simulink model "Forward_and_inverse_Both"  (R2024b)
settings: Solver=VariableStepAuto  StartTime=0.0  StopTime=7  MaxStep=0.005  RelTol=1e-3
model workspace: external: MATLAB File D:\OneDrive - itc.edu.kh\V4_robot_arm\Import_arm6\Test_Assembly_DataFile.m (data not in the file)
values from neighbouring files (symbols this model uses):
  Reach_max = max(REACH_MAX)    [Workspace_sample.m]
  Reach_min = max(REACH_MIN)    [Workspace_sample.m]
undefined symbols (not defined in the file or in its folder): DiscIntNeverNeededParam, initialPose, maxAngularAcc, maxAngularVel, maxLinearAcc, maxLinearVel, poseTol, smiData, Ts, wps1, X, Y, Z
libraries: sm_lib x140, nesl_utility x52, stmnucleolib x12, simulink x4, vrlib x2, vexcommonlib x2, robotcorelib x2
(part 3 of 6)

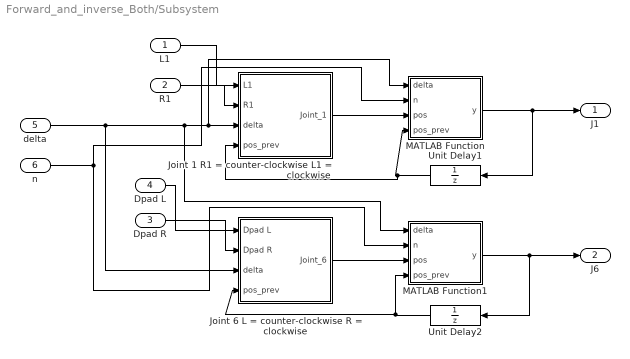
== system Forward_and_inverse_Both/Subsystem ==
  L1 : Inport
  R1 : Inport  Port=2
  Dpad R : Inport  Port=3
  Dpad L : Inport  Port=4
  delta : Inport  Port=5
  n : Inport  Port=6
  Joint 1 R1 = counter-clockwise L1 = clockwise : Subsystem
  Joint 6 L = counter-clockwise R = clockwise : Subsystem
  MATLAB Function : MATLAB Function  TreatAsAtomicUnit=on
  MATLAB Function1 : MATLAB Function  TreatAsAtomicUnit=on
  Unit Delay1 : UnitDelay  SampleTime=-1  HasFrameUpgradeWarning=on
  Unit Delay2 : UnitDelay  SampleTime=-1  HasFrameUpgradeWarning=on
  J1 : Outport
  J6 : Outport  Port=2
  wires:
  delta/1 -> Joint 6 L = counter-clockwise R = clockwise/3(delta), MATLAB Function1/1(delta), MATLAB Function/1(delta), Joint 1 R1 = counter-clockwise L1 = clockwise/3(delta)
  R1/1 -> Joint 1 R1 = counter-clockwise L1 = clockwise/2(R1)
  L1/1 -> Joint 1 R1 = counter-clockwise L1 = clockwise/1(L1)
  Dpad L/1 -> Joint 6 L = counter-clockwise R = clockwise/1(Dpad L)
  Dpad R/1 -> Joint 6 L = counter-clockwise R = clockwise/2(Dpad R)
  n/1 -> MATLAB Function1/2(n), MATLAB Function/2(n)
  Unit Delay1/1 -> Joint 1 R1 = counter-clockwise L1 = clockwise/4(pos_prev), MATLAB Function/4(pos_prev)
  Joint 1 R1 = counter-clockwise L1 = clockwise/1(Joint_1) -> MATLAB Function/3(pos)
  MATLAB Function/1(y) -> J1/1, Unit Delay1/1
  MATLAB Function1/1(y) -> J6/1, Unit Delay2/1
  Joint 6 L = counter-clockwise R = clockwise/1(Joint_6) -> MATLAB Function1/3(pos)
  Unit Delay2/1 -> Joint 6 L = counter-clockwise R = clockwise/4(pos_prev), MATLAB Function1/4(pos_prev)

== system Forward_and_inverse_Both/Subsystem1 ==
  Desired Position : Inport
  MATLAB Function : MATLAB Function  TreatAsAtomicUnit=on
  reset : Constant  Value=0
  speedMode : Constant  Value=0  OutDataTypeStr=int16
  stop : Constant  Value=0  OutDataTypeStr=int16
  voltageMode : Constant  Value=0
  Output to CAN : Outport
  wires:
  reset/1 -> MATLAB Function/4(reset)
  Desired Position/1 -> MATLAB Function/1(goal)
  speedMode/1 -> MATLAB Function/2(speedMode)
  stop/1 -> MATLAB Function/3(stop)
  MATLAB Function/1(Msg) -> Output to CAN/1
  voltageMode/1 -> MATLAB Function/5(voltageMode)

== system Forward_and_inverse_Both/Subsystem10 ==
  data : Inport
  MATLAB Function : MATLAB Function  TreatAsAtomicUnit=on
  Terminator : Terminator
  position : Outport
  wires:
  MATLAB Function/2(speed) -> Terminator/1
  MATLAB Function/1(position) -> position/1
  data/1 -> MATLAB Function/1(data)

== system Forward_and_inverse_Both/Subsystem11 ==
  data : Inport
  MATLAB Function : MATLAB Function  TreatAsAtomicUnit=on
  Terminator : Terminator
  position : Outport
  wires:
  MATLAB Function/2(speed) -> Terminator/1
  MATLAB Function/1(position) -> position/1
  data/1 -> MATLAB Function/1(data)

== system Forward_and_inverse_Both/Subsystem12 ==
  data : Inport
  MATLAB Function : MATLAB Function  TreatAsAtomicUnit=on
  Terminator : Terminator
  position : Outport
  wires:
  MATLAB Function/2(speed) -> Terminator/1
  MATLAB Function/1(position) -> position/1
  data/1 -> MATLAB Function/1(data)

== system Forward_and_inverse_Both/Subsystem13 ==
  q1 : Inport
  Constant1 : Constant
  Define Relative angle1 : MATLAB Function  TreatAsAtomicUnit=on
  Ground : Ground
  Ground1 : Ground
  angle : Outport
  wires:
  Ground/1 -> Define Relative angle1/1(initialPose)
  Define Relative angle1/1(angle) -> angle/1
  Constant1/1 -> Define Relative angle1/4(status)
  Ground1/1 -> Define Relative angle1/2(reset_angle)
  q1/1 -> Define Relative angle1/3(rawangle)

== system Forward_and_inverse_Both/Subsystem14 ==
  q1 : Inport
  Constant1 : Constant
  Define Relative angle1 : MATLAB Function  TreatAsAtomicUnit=on
  Ground : Ground
  Ground1 : Ground
  angle : Outport
  wires:
  Ground/1 -> Define Relative angle1/1(initialPose)
  Define Relative angle1/1(angle) -> angle/1
  Constant1/1 -> Define Relative angle1/4(status)
  Ground1/1 -> Define Relative angle1/2(reset_angle)
  q1/1 -> Define Relative angle1/3(rawangle)

== system Forward_and_inverse_Both/Subsystem15 ==
  q1 : Inport
  Constant1 : Constant
  Define Relative angle1 : MATLAB Function  TreatAsAtomicUnit=on
  Ground : Ground
  Ground1 : Ground
  angle : Outport
  wires:
  Ground/1 -> Define Relative angle1/1(initialPose)
  Define Relative angle1/1(angle) -> angle/1
  Constant1/1 -> Define Relative angle1/4(status)
  Ground1/1 -> Define Relative angle1/2(reset_angle)
  q1/1 -> Define Relative angle1/3(rawangle)

== system Forward_and_inverse_Both/Subsystem16 ==
  q1 : Inport
  Constant1 : Constant
  Define Relative angle1 : MATLAB Function  TreatAsAtomicUnit=on
  Ground : Ground
  Ground1 : Ground
  angle : Outport
  wires:
  q1/1 -> Define Relative angle1/3(rawangle)
  Ground1/1 -> Define Relative angle1/2(reset_angle)
  Constant1/1 -> Define Relative angle1/4(status)
  Define Relative angle1/1(angle) -> angle/1
  Ground/1 -> Define Relative angle1/1(initialPose)

== system Forward_and_inverse_Both/Subsystem17 ==
  q1 : Inport
  Constant1 : Constant
  Define Relative angle : MATLAB Function  TreatAsAtomicUnit=on
  Ground : Ground
  Ground1 : Ground
  angle : Outport
  wires:
  Ground/1 -> Define Relative angle/1(initialPose)
  Define Relative angle/1(angle) -> angle/1
  Constant1/1 -> Define Relative angle/4(status)
  Ground1/1 -> Define Relative angle/2(reset_angle)
  q1/1 -> Define Relative angle/3(rawangle)

== system Forward_and_inverse_Both/Subsystem18 ==
  q1 : Inport
  Constant1 : Constant
  Define Relative angle1 : MATLAB Function  TreatAsAtomicUnit=on
  Ground : Ground
  Ground1 : Ground
  angle : Outport
  wires:
  Ground/1 -> Define Relative angle1/1(initialPose)
  Define Relative angle1/1(angle) -> angle/1
  Constant1/1 -> Define Relative angle1/4(status)
  Ground1/1 -> Define Relative angle1/2(reset_angle)
  q1/1 -> Define Relative angle1/3(rawangle)

== system Forward_and_inverse_Both/Subsystem19 ==
  Joystick Input : vrlib/Joystick Input  joyid=1  adjustports=on  forcefeed=off
  Use this block for PS4 controller : vexcommonlib/Gamepad Simulator  WhichPad=XBox Gamepad  JoyId=1  BlockPlatform=vexarmcortex
      settings: LibrarySourceBlock=vexarmcortexlib/Utilities/Gamepad Simulator
  Out1 : Outport
  D5_up : Outport  Port=2
  D6_up : Outport  Port=3
  D_right : Outport  Port=4
  D_left : Outport  Port=5
  D8_left : Outport  Port=6
  D8_down : Outport  Port=7
  D8_right : Outport  Port=8
  wires:
  Use this block for PS4 controller/12 -> D8_left/1
  Use this block for PS4 controller/10 -> D8_down/1
  Joystick Input/1 -> Out1/1
  Use this block for PS4 controller/7 -> D6_up/1
  Use this block for PS4 controller/14 -> D_right/1  "D_right"
  Use this block for PS4 controller/16 -> D_left/1  "D_left"
  Use this block for PS4 controller/5 -> D5_up/1
  Use this block for PS4 controller/11 -> D8_right/1

== system Forward_and_inverse_Both/Subsystem2 ==
  Desired Position : Inport
  MATLAB Function : MATLAB Function  TreatAsAtomicUnit=on
  reset : Constant  Value=0
  speedMode : Constant  Value=0  OutDataTypeStr=int16
  stop : Constant  Value=0  OutDataTypeStr=int16
  voltageMode : Constant  Value=0
  Output to CAN : Outport
  wires:
  reset/1 -> MATLAB Function/4(reset)
  Desired Position/1 -> MATLAB Function/1(goal)
  speedMode/1 -> MATLAB Function/2(speedMode)
  stop/1 -> MATLAB Function/3(stop)
  MATLAB Function/1(Msg) -> Output to CAN/1
  voltageMode/1 -> MATLAB Function/5(voltageMode)

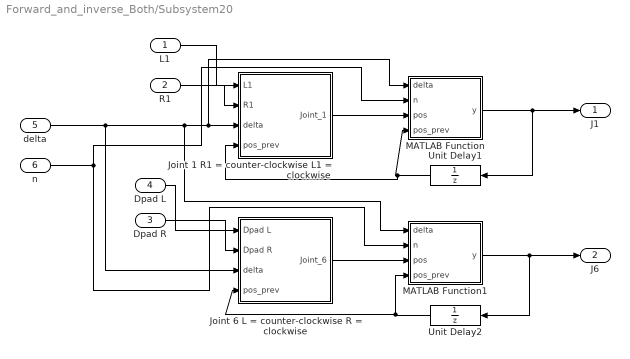
== system Forward_and_inverse_Both/Subsystem20 ==
  L1 : Inport
  R1 : Inport  Port=2
  Dpad R : Inport  Port=3
  Dpad L : Inport  Port=4
  delta : Inport  Port=5
  n : Inport  Port=6
  Joint 1 R1 = counter-clockwise L1 = clockwise : Subsystem
  Joint 6 L = counter-clockwise R = clockwise : Subsystem
  MATLAB Function : MATLAB Function  TreatAsAtomicUnit=on
  MATLAB Function1 : MATLAB Function  TreatAsAtomicUnit=on
  Unit Delay1 : UnitDelay  SampleTime=-1  HasFrameUpgradeWarning=on
  Unit Delay2 : UnitDelay  SampleTime=-1  HasFrameUpgradeWarning=on
  J1 : Outport
  J6 : Outport  Port=2
  wires:
  delta/1 -> Joint 6 L = counter-clockwise R = clockwise/3(delta), MATLAB Function1/1(delta), MATLAB Function/1(delta), Joint 1 R1 = counter-clockwise L1 = clockwise/3(delta)
  R1/1 -> Joint 1 R1 = counter-clockwise L1 = clockwise/2(R1)
  L1/1 -> Joint 1 R1 = counter-clockwise L1 = clockwise/1(L1)
  Dpad L/1 -> Joint 6 L = counter-clockwise R = clockwise/1(Dpad L)
  Dpad R/1 -> Joint 6 L = counter-clockwise R = clockwise/2(Dpad R)
  n/1 -> MATLAB Function1/2(n), MATLAB Function/2(n)
  Unit Delay1/1 -> Joint 1 R1 = counter-clockwise L1 = clockwise/4(pos_prev), MATLAB Function/4(pos_prev)
  Joint 1 R1 = counter-clockwise L1 = clockwise/1(Joint_1) -> MATLAB Function/3(pos)
  MATLAB Function/1(y) -> J1/1, Unit Delay1/1
  MATLAB Function1/1(y) -> J6/1, Unit Delay2/1
  Joint 6 L = counter-clockwise R = clockwise/1(Joint_6) -> MATLAB Function1/3(pos)
  Unit Delay2/1 -> Joint 6 L = counter-clockwise R = clockwise/4(pos_prev), MATLAB Function1/4(pos_prev)

== system Forward_and_inverse_Both/Subsystem21 ==
  Joystick Input : vrlib/Joystick Input  joyid=1  adjustports=on  forcefeed=off
  Use this block for PS4 controller : vexcommonlib/Gamepad Simulator  WhichPad=XBox Gamepad  JoyId=1  BlockPlatform=vexarmcortex
  Out1 : Outport
  D5_up : Outport  Port=2
  D6_up : Outport  Port=3
  D_right : Outport  Port=4
  D_left : Outport  Port=5
  D8_left : Outport  Port=6
  D8_down : Outport  Port=7
  D8_right : Outport  Port=8
  wires:
  Use this block for PS4 controller/12 -> D8_left/1
  Use this block for PS4 controller/10 -> D8_down/1
  Joystick Input/1 -> Out1/1
  Use this block for PS4 controller/7 -> D6_up/1
  Use this block for PS4 controller/14 -> D_right/1  "D_right"
  Use this block for PS4 controller/16 -> D_left/1  "D_left"
  Use this block for PS4 controller/5 -> D5_up/1
  Use this block for PS4 controller/11 -> D8_right/1

== system Forward_and_inverse_Both/Subsystem24 ==
  q1 : Inport
  Constant1 : Constant
  Define Relative angle1 : MATLAB Function  TreatAsAtomicUnit=on
  Ground : Ground
  Ground1 : Ground
  angle : Outport
  wires:
  q1/1 -> Define Relative angle1/3(rawangle)
  Ground1/1 -> Define Relative angle1/2(reset_angle)
  Constant1/1 -> Define Relative angle1/4(status)
  Define Relative angle1/1(angle) -> angle/1
  Ground/1 -> Define Relative angle1/1(initialPose)

== system Forward_and_inverse_Both/Subsystem25 ==
  q1 : Inport
  Constant1 : Constant
  Define Relative angle : MATLAB Function  TreatAsAtomicUnit=on
  Ground : Ground
  Ground1 : Ground
  angle : Outport
  wires:
  Ground/1 -> Define Relative angle/1(initialPose)
  Define Relative angle/1(angle) -> angle/1
  Constant1/1 -> Define Relative angle/4(status)
  Ground1/1 -> Define Relative angle/2(reset_angle)
  q1/1 -> Define Relative angle/3(rawangle)

== system Forward_and_inverse_Both/Subsystem3 ==
  Desired Position : Inport
  MATLAB Function : MATLAB Function  TreatAsAtomicUnit=on
  reset : Constant  Value=0
  speedMode : Constant  Value=0  OutDataTypeStr=int16
  stop : Constant  Value=0  OutDataTypeStr=int16
  voltageMode : Constant  Value=0
  Output to CAN : Outport
  wires:
  reset/1 -> MATLAB Function/4(reset)
  Desired Position/1 -> MATLAB Function/1(goal)
  speedMode/1 -> MATLAB Function/2(speedMode)
  stop/1 -> MATLAB Function/3(stop)
  MATLAB Function/1(Msg) -> Output to CAN/1
  voltageMode/1 -> MATLAB Function/5(voltageMode)

== system Forward_and_inverse_Both/Subsystem4 ==
  Desired Position : Inport
  MATLAB Function : MATLAB Function  TreatAsAtomicUnit=on
  reset : Constant  Value=0
  speedMode : Constant  Value=0  OutDataTypeStr=int16
  stop : Constant  Value=0  OutDataTypeStr=int16
  voltageMode : Constant  Value=0
  Output to CAN : Outport
  wires:
  reset/1 -> MATLAB Function/4(reset)
  Desired Position/1 -> MATLAB Function/1(goal)
  speedMode/1 -> MATLAB Function/2(speedMode)
  stop/1 -> MATLAB Function/3(stop)
  MATLAB Function/1(Msg) -> Output to CAN/1
  voltageMode/1 -> MATLAB Function/5(voltageMode)

== system Forward_and_inverse_Both/Subsystem5 ==
  Desired Position : Inport
  MATLAB Function : MATLAB Function  TreatAsAtomicUnit=on
  reset : Constant  Value=0
  speedMode : Constant  Value=0  OutDataTypeStr=int16
  stop : Constant  Value=0  OutDataTypeStr=int16
  voltageMode : Constant  Value=0
  Output to CAN : Outport
  wires:
  reset/1 -> MATLAB Function/4(reset)
  Desired Position/1 -> MATLAB Function/1(goal)
  speedMode/1 -> MATLAB Function/2(speedMode)
  stop/1 -> MATLAB Function/3(stop)
  MATLAB Function/1(Msg) -> Output to CAN/1
  voltageMode/1 -> MATLAB Function/5(voltageMode)

== system Forward_and_inverse_Both/Subsystem6 ==
  Desired Position : Inport
  MATLAB Function : MATLAB Function  TreatAsAtomicUnit=on
  reset : Constant  Value=0
  speedMode : Constant  Value=0  OutDataTypeStr=int16
  stop : Constant  Value=0  OutDataTypeStr=int16
  voltageMode : Constant  Value=0
  Output to CAN : Outport
  wires:
  reset/1 -> MATLAB Function/4(reset)
  Desired Position/1 -> MATLAB Function/1(goal)
  speedMode/1 -> MATLAB Function/2(speedMode)
  stop/1 -> MATLAB Function/3(stop)
  MATLAB Function/1(Msg) -> Output to CAN/1
  voltageMode/1 -> MATLAB Function/5(voltageMode)

== system Forward_and_inverse_Both/Subsystem7 ==
  data : Inport
  MATLAB Function : MATLAB Function  TreatAsAtomicUnit=on
  Terminator : Terminator
  position : Outport
  wires:
  MATLAB Function/2(speed) -> Terminator/1
  MATLAB Function/1(position) -> position/1
  data/1 -> MATLAB Function/1(data)

== system Forward_and_inverse_Both/Subsystem8 ==
  data : Inport
  MATLAB Function : MATLAB Function  TreatAsAtomicUnit=on
  Terminator : Terminator
  position : Outport
  wires:
  MATLAB Function/2(speed) -> Terminator/1
  MATLAB Function/1(position) -> position/1
  data/1 -> MATLAB Function/1(data)

== system Forward_and_inverse_Both/Subsystem9 ==
  data : Inport
  MATLAB Function : MATLAB Function  TreatAsAtomicUnit=on
  Terminator : Terminator
  position : Outport
  wires:
  MATLAB Function/2(speed) -> Terminator/1
  MATLAB Function/1(position) -> position/1
  data/1 -> MATLAB Function/1(data)

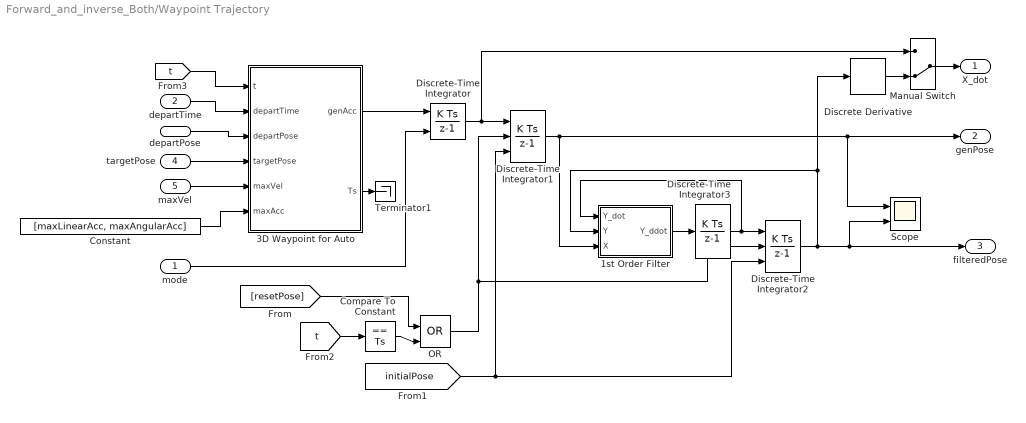
== system Forward_and_inverse_Both/Waypoint Trajectory ==
  mode : Inport
  departTime : Inport  Port=2
  departPose : Inport  Port=3
  targetPose : Inport  Port=4
  maxVel : Inport  Port=5
  1st Order Filter : MATLAB Function  TreatAsAtomicUnit=on
  3D Waypoint for Auto : MATLAB Function  TreatAsAtomicUnit=on
  Compare To Constant : simulink/Logic and Bit Operations/Compare To Constant  relop===  const=Ts  OutDataTypeStr=boolean
  Constant : Constant  Value=[maxLinearAcc, maxAngularAcc]
  Discrete Derivative : simulink/Discrete/Discrete Derivative  gainval=1.0  ICPrevScaledInput=0.0  OutMin=[]  OutMax=[]  OutDataType=fixdt(1, 16)  OutScaling=2^-10  DoSatur=off
  Discrete-Time Integrator : DiscreteIntegrator  ExternalReset=falling  InitialCondition=[0;0;0;0]  SampleTime=-1  ICPrevOutput=DiscIntNeverNeededParam  ICPrevScaledInput=DiscIntNeverNeededParam
  Discrete-Time Integrator1 : DiscreteIntegrator  ExternalReset=rising  InitialConditionSource=external  InitialCondition=[0;0;0;0]  SampleTime=-1  ICPrevOutput=DiscIntNeverNeededParam  ICPrevScaledInput=DiscIntNeverNeededParam
  Discrete-Time Integrator2 : DiscreteIntegrator  ExternalReset=rising  InitialConditionSource=external  InitialCondition=[0;0;0;0]  SampleTime=-1  ICPrevOutput=DiscIntNeverNeededParam  ICPrevScaledInput=DiscIntNeverNeededParam
  Discrete-Time Integrator3 : DiscreteIntegrator  InitialCondition=[0;0;0;0]  SampleTime=-1  ICPrevOutput=DiscIntNeverNeededParam  ICPrevScaledInput=DiscIntNeverNeededParam
  Manual Switch : ManualSwitch  CurrentSetting=0
  OR : Logic  Operator=OR  IconShape=distinctive  AllPortsSameDT=off  OutDataTypeStr=boolean
  Scope : Scope  NumInputPorts=2
  Terminator1 : Terminator
  X_dot : Outport
  genPose : Outport  Port=2
  filteredPose : Outport  Port=3
  wires:
  Constant/1 -> 3D Waypoint for Auto/6(maxAcc)
  targetPose/1 -> 3D Waypoint for Auto/4(targetPose)
  maxVel/1 -> 3D Waypoint for Auto/5(maxVel)
  departTime/1 -> 3D Waypoint for Auto/2(departTime)
  [t] -> 3D Waypoint for Auto/1(t)
  departPose/1 -> 3D Waypoint for Auto/3(departPose)
  3D Waypoint for Auto/2(Ts) -> Terminator1/1
  Discrete-Time Integrator/1 -> Discrete-Time Integrator1/1, Manual Switch/1
  [t] -> Compare To Constant/1
  [resetPose] -> OR/1
  Compare To Constant/1 -> OR/2
  3D Waypoint for Auto/1(genAcc) -> Discrete-Time Integrator/1
  mode/1 -> Discrete-Time Integrator/2
  OR/1 -> Discrete-Time Integrator2/2, Discrete-Time Integrator1/2
  [initialPose] -> Discrete-Time Integrator1/3, Discrete-Time Integrator2/3
  Discrete-Time Integrator1/1 -> Scope/1, genPose/1, 1st Order Filter/3(X)
  1st Order Filter/1(Y_ddot) -> Discrete-Time Integrator3/1
  Discrete-Time Integrator2/1 -> Scope/2, filteredPose/1, Discrete Derivative/1, 1st Order Filter/2(Y)
  Discrete Derivative/1 -> Manual Switch/2
  Manual Switch/1 -> X_dot/1
  Discrete-Time Integrator3/1 -> 1st Order Filter/1(Y_dot), Discrete-Time Integrator2/1

== system Forward_and_inverse_Both/6 DOF robot arm/Base_2_RIGID ==
  ReferenceFrame : sm_lib/Frames and Transforms/Reference Frame
  Solid : sm_lib/Body Elements/File Solid  ExtGeomFileName=C:\Drive D\Material\DC LAB\simscape\simscape\Solidworks FIle\Base_Default_sldprt.STEP  UnitType=Custom  ExtGeomFileUnits=m  StepReaderType=HEX  ExportConvexHullGeometry=off  InertiaType=Custom  BasedOnType=DensityFromFile  Density=1000  DensityUnits=kg/m^3  Mass=smiData.Solid(1).mass  MassUnits=kg  CenterOfMass=smiData.Solid(1).CoM  CenterOfMassUnits=mm  MomentsOfInertia=smiData.Solid(1).MoI  MomentsOfInertiaUnits=kg*mm^2  ProductsOfInertia=smiData.Solid(1).PoI  ProductsOfInertiaUnits=kg*mm^2  GraphicType=FromGeometry  MarkerShape=Sphere  MarkerSize=10  GraphicVisPropType=SimpleVisualProperties  GraphicDiffuseColor=smiData.Solid(1).color  GraphicOpacity=smiData.Solid(1).opacity  GraphicSpecularColor=[0.5 0.5 0.5 1.0]  GraphicAmbientColor=[0.15 0.15 0.15 1.0]  GraphicEmissiveColor=[0.0 0.0 0.0 1.0]  GraphicShininess=75  DoExposeReferenceFrame=on  SerializedFrames=<Frames/>
  Transform : sm_lib/Frames and Transforms/Rigid Transform  RotationMethod=ArbitraryAxis  FollAlignAxisA=+X  BaseAlignAxisA=+Y  FollAlignAxisB=+Y  BaseAlignAxisB=+Z  RotationStandardAxis=+Z  RotationAngle=smiData.RigidTransform(5).angle  RotationAngleUnits=rad  RotationArbitraryAxis=smiData.RigidTransform(5).axis  RotationSequenceAxes=FollowerAxes  RotationSequence=XYX  RotationSequenceAngles=[0 0 0]  RotationSequenceAnglesUnits=deg  RotationMatrix=[1 0 0; 0 1 0; 0 0 1]  Quaternion=[1 0 0 0]  TranslationMethod=Cartesian  TranslationCartesianOffset=smiData.RigidTransform(5).translation  TranslationCartesianOffsetUnits=m  TranslationStandardAxis=+Z  TranslationStandardOffset=0  TranslationStandardOffsetUnits=m  TranslationROffset=0  TranslationROffsetUnits=m  TranslationThetaOffset=0  TranslationThetaOffsetUnits=deg  TranslationZOffset=0  TranslationZOffsetUnits=m
  F1 : PMIOPort  Side=Left
  F : PMIOPort  Port=2  Side=Right
  connections:
  Solid/RConn1 -- ReferenceFrame/RConn1 -- Transform/LConn1 -- F1/RConn1
  Transform/RConn1 -- F/RConn1

== system Forward_and_inverse_Both/6 DOF robot arm/L1_v2_1_RIGID ==
  ReferenceFrame : sm_lib/Frames and Transforms/Reference Frame
  Solid : sm_lib/Body Elements/File Solid  ExtGeomFileName=C:\Drive D\Material\DC LAB\simscape\simscape\Solidworks FIle\L1_v2_Default_sldprt.STEP  UnitType=Custom  ExtGeomFileUnits=m  StepReaderType=HEX  ExportConvexHullGeometry=off  InertiaType=Custom  BasedOnType=DensityFromFile  Density=1000  DensityUnits=kg/m^3  Mass=smiData.Solid(5).mass  MassUnits=kg  CenterOfMass=smiData.Solid(5).CoM  CenterOfMassUnits=mm  MomentsOfInertia=smiData.Solid(5).MoI  MomentsOfInertiaUnits=kg*mm^2  ProductsOfInertia=smiData.Solid(5).PoI  ProductsOfInertiaUnits=kg*mm^2  GraphicType=FromGeometry  MarkerShape=Sphere  MarkerSize=10  GraphicVisPropType=SimpleVisualProperties  GraphicDiffuseColor=[0.0 0.8 0.8]  GraphicOpacity=smiData.Solid(5).opacity  GraphicSpecularColor=[0.5 0.5 0.5 1.0]  GraphicAmbientColor=[0.15 0.15 0.15 1.0]  GraphicEmissiveColor=[0.0 0.0 0.0 1.0]  GraphicShininess=75  DoExposeReferenceFrame=on  SerializedFrames=<Frames/>
  Transform : sm_lib/Frames and Transforms/Rigid Transform  RotationMethod=ArbitraryAxis  FollAlignAxisA=+X  BaseAlignAxisA=+Y  FollAlignAxisB=+Y  BaseAlignAxisB=+Z  RotationStandardAxis=+Z  RotationAngle=smiData.RigidTransform(6).angle  RotationAngleUnits=rad  RotationArbitraryAxis=smiData.RigidTransform(6).axis  RotationSequenceAxes=FollowerAxes  RotationSequence=XYX  RotationSequenceAngles=[0 0 0]  RotationSequenceAnglesUnits=deg  RotationMatrix=[1 0 0; 0 1 0; 0 0 1]  Quaternion=[1 0 0 0]  TranslationMethod=Cartesian  TranslationCartesianOffset=smiData.RigidTransform(6).translation  TranslationCartesianOffsetUnits=m  TranslationStandardAxis=+Z  TranslationStandardOffset=0  TranslationStandardOffsetUnits=m  TranslationROffset=0  TranslationROffsetUnits=m  TranslationThetaOffset=0  TranslationThetaOffsetUnits=deg  TranslationZOffset=0  TranslationZOffsetUnits=m
  Transform1 : sm_lib/Frames and Transforms/Rigid Transform  RotationMethod=ArbitraryAxis  FollAlignAxisA=+X  BaseAlignAxisA=+Y  FollAlignAxisB=+Y  BaseAlignAxisB=+Z  RotationStandardAxis=+Z  RotationAngle=smiData.RigidTransform(7).angle  RotationAngleUnits=rad  RotationArbitraryAxis=smiData.RigidTransform(7).axis  RotationSequenceAxes=FollowerAxes  RotationSequence=XYX  RotationSequenceAngles=[0 0 0]  RotationSequenceAnglesUnits=deg  RotationMatrix=[1 0 0; 0 1 0; 0 0 1]  Quaternion=[1 0 0 0]  TranslationMethod=Cartesian  TranslationCartesianOffset=smiData.RigidTransform(7).translation  TranslationCartesianOffsetUnits=m  TranslationStandardAxis=+Z  TranslationStandardOffset=0  TranslationStandardOffsetUnits=m  TranslationROffset=0  TranslationROffsetUnits=m  TranslationThetaOffset=0  TranslationThetaOffsetUnits=deg  TranslationZOffset=0  TranslationZOffsetUnits=m
  F : PMIOPort  Side=Left
  F1 : PMIOPort  Port=2  Side=Right
  connections:
  Solid/RConn1 -- ReferenceFrame/RConn1 -- Transform/LConn1 -- Transform1/LConn1
  Transform/RConn1 -- F/RConn1
  Transform1/RConn1 -- F1/RConn1

== system Forward_and_inverse_Both/6 DOF robot arm/L2_v4_1_RIGID ==
  ReferenceFrame : sm_lib/Frames and Transforms/Reference Frame
  Solid : sm_lib/Body Elements/File Solid  ExtGeomFileName=C:\Drive D\Material\DC LAB\simscape\simscape\Solidworks FIle\L2_v4_Default_sldprt.STEP  UnitType=Custom  ExtGeomFileUnits=m  StepReaderType=HEX  ExportConvexHullGeometry=off  InertiaType=Custom  BasedOnType=DensityFromFile  Density=1000  DensityUnits=kg/m^3  Mass=smiData.Solid(3).mass  MassUnits=kg  CenterOfMass=smiData.Solid(3).CoM  CenterOfMassUnits=mm  MomentsOfInertia=smiData.Solid(3).MoI  MomentsOfInertiaUnits=kg*mm^2  ProductsOfInertia=smiData.Solid(3).PoI  ProductsOfInertiaUnits=kg*mm^2  GraphicType=FromGeometry  MarkerShape=Sphere  MarkerSize=10  GraphicVisPropType=SimpleVisualProperties  GraphicDiffuseColor=[0.0 0.8 0.8]  GraphicOpacity=smiData.Solid(3).opacity  GraphicSpecularColor=[0.5 0.5 0.5 1.0]  GraphicAmbientColor=[0.15 0.15 0.15 1.0]  GraphicEmissiveColor=[0.0 0.0 0.0 1.0]  GraphicShininess=75  DoExposeReferenceFrame=on  SerializedFrames=<Frames/>
  Transform : sm_lib/Frames and Transforms/Rigid Transform  RotationMethod=ArbitraryAxis  FollAlignAxisA=+X  BaseAlignAxisA=+Y  FollAlignAxisB=+Y  BaseAlignAxisB=+Z  RotationStandardAxis=+Z  RotationAngle=smiData.RigidTransform(8).angle  RotationAngleUnits=rad  RotationArbitraryAxis=smiData.RigidTransform(8).axis  RotationSequenceAxes=FollowerAxes  RotationSequence=XYX  RotationSequenceAngles=[0 0 0]  RotationSequenceAnglesUnits=deg  RotationMatrix=[1 0 0; 0 1 0; 0 0 1]  Quaternion=[1 0 0 0]  TranslationMethod=Cartesian  TranslationCartesianOffset=smiData.RigidTransform(8).translation  TranslationCartesianOffsetUnits=m  TranslationStandardAxis=+Z  TranslationStandardOffset=0  TranslationStandardOffsetUnits=m  TranslationROffset=0  TranslationROffsetUnits=m  TranslationThetaOffset=0  TranslationThetaOffsetUnits=deg  TranslationZOffset=0  TranslationZOffsetUnits=m
  Transform1 : sm_lib/Frames and Transforms/Rigid Transform  RotationMethod=ArbitraryAxis  FollAlignAxisA=+X  BaseAlignAxisA=+Y  FollAlignAxisB=+Y  BaseAlignAxisB=+Z  RotationStandardAxis=+Z  RotationAngle=smiData.RigidTransform(11).angle  RotationAngleUnits=rad  RotationArbitraryAxis=smiData.RigidTransform(11).axis  RotationSequenceAxes=FollowerAxes  RotationSequence=XYX  RotationSequenceAngles=[0 0 0]  RotationSequenceAnglesUnits=deg  RotationMatrix=[1 0 0; 0 1 0; 0 0 1]  Quaternion=[1 0 0 0]  TranslationMethod=Cartesian  TranslationCartesianOffset=smiData.RigidTransform(11).translation  TranslationCartesianOffsetUnits=m  TranslationStandardAxis=+Z  TranslationStandardOffset=0  TranslationStandardOffsetUnits=m  TranslationROffset=0  TranslationROffsetUnits=m  TranslationThetaOffset=0  TranslationThetaOffsetUnits=deg  TranslationZOffset=0  TranslationZOffsetUnits=m
  F : PMIOPort  Side=Left
  F1 : PMIOPort  Port=2  Side=Right
  connections:
  Solid/RConn1 -- ReferenceFrame/RConn1 -- Transform/LConn1 -- Transform1/LConn1
  Transform/RConn1 -- F/RConn1
  Transform1/RConn1 -- F1/RConn1

== system Forward_and_inverse_Both/6 DOF robot arm/L6_2_RIGID ==
  ReferenceFrame : sm_lib/Frames and Transforms/Reference Frame
  Solid : sm_lib/Body Elements/File Solid  ExtGeomFileName=C:\Drive D\Material\DC LAB\simscape\simscape\Solidworks FIle\L6_Default_sldprt.STEP  UnitType=Custom  ExtGeomFileUnits=m  StepReaderType=HEX  ExportConvexHullGeometry=off  InertiaType=Custom  BasedOnType=DensityFromFile  Density=1000  DensityUnits=kg/m^3  Mass=smiData.Solid(7).mass  MassUnits=kg  CenterOfMass=smiData.Solid(7).CoM  CenterOfMassUnits=mm  MomentsOfInertia=smiData.Solid(7).MoI  MomentsOfInertiaUnits=kg*mm^2  ProductsOfInertia=smiData.Solid(7).PoI  ProductsOfInertiaUnits=kg*mm^2  GraphicType=FromGeometry  MarkerShape=Sphere  MarkerSize=10  GraphicVisPropType=SimpleVisualProperties  GraphicDiffuseColor=[0.0 0.8 0.8]  GraphicOpacity=smiData.Solid(7).opacity  GraphicSpecularColor=[0.5 0.5 0.5 1.0]  GraphicAmbientColor=[0.15 0.15 0.15 1.0]  GraphicEmissiveColor=[0.0 0.0 0.0 1.0]  GraphicShininess=75  DoExposeReferenceFrame=on  SerializedFrames=<Frames/>
  Transform : sm_lib/Frames and Transforms/Rigid Transform  RotationMethod=ArbitraryAxis  FollAlignAxisA=+X  BaseAlignAxisA=+Y  FollAlignAxisB=+Y  BaseAlignAxisB=+Z  RotationStandardAxis=+Z  RotationAngle=smiData.RigidTransform(10).angle  RotationAngleUnits=rad  RotationArbitraryAxis=smiData.RigidTransform(10).axis  RotationSequenceAxes=FollowerAxes  RotationSequence=XYX  RotationSequenceAngles=[0 0 0]  RotationSequenceAnglesUnits=deg  RotationMatrix=[1 0 0; 0 1 0; 0 0 1]  Quaternion=[1 0 0 0]  TranslationMethod=Cartesian  TranslationCartesianOffset=smiData.RigidTransform(10).translation  TranslationCartesianOffsetUnits=m  TranslationStandardAxis=+Z  TranslationStandardOffset=0  TranslationStandardOffsetUnits=m  TranslationROffset=0  TranslationROffsetUnits=m  TranslationThetaOffset=0  TranslationThetaOffsetUnits=deg  TranslationZOffset=0  TranslationZOffsetUnits=m
  F : PMIOPort  Side=Left
  connections:
  Solid/RConn1 -- ReferenceFrame/RConn1 -- Transform/LConn1
  Transform/RConn1 -- F/RConn1

== system Forward_and_inverse_Both/6 DOF robot arm/Link3_v2_1_RIGID ==
  ReferenceFrame : sm_lib/Frames and Transforms/Reference Frame
  Solid : sm_lib/Body Elements/File Solid  ExtGeomFileName=C:\Drive D\Material\DC LAB\simscape\simscape\Solidworks FIle\Link3_v2_Default_sldprt.STEP  UnitType=Custom  ExtGeomFileUnits=m  StepReaderType=HEX  ExportConvexHullGeometry=off  InertiaType=Custom  BasedOnType=DensityFromFile  Density=1000  DensityUnits=kg/m^3  Mass=smiData.Solid(2).mass  MassUnits=kg  CenterOfMass=smiData.Solid(2).CoM  CenterOfMassUnits=mm  MomentsOfInertia=smiData.Solid(2).MoI  MomentsOfInertiaUnits=kg*mm^2  ProductsOfInertia=smiData.Solid(2).PoI  ProductsOfInertiaUnits=kg*mm^2  GraphicType=FromGeometry  MarkerShape=Sphere  MarkerSize=10  GraphicVisPropType=SimpleVisualProperties  GraphicDiffuseColor=[0.0 0.8 0.8]  GraphicOpacity=smiData.Solid(2).opacity  GraphicSpecularColor=[0.5 0.5 0.5 1.0]  GraphicAmbientColor=[0.15 0.15 0.15 1.0]  GraphicEmissiveColor=[0.0 0.0 0.0 1.0]  GraphicShininess=75  DoExposeReferenceFrame=on  SerializedFrames=<Frames/>
  Transform : sm_lib/Frames and Transforms/Rigid Transform  RotationMethod=ArbitraryAxis  FollAlignAxisA=+X  BaseAlignAxisA=+Y  FollAlignAxisB=+Y  BaseAlignAxisB=+Z  RotationStandardAxis=+Z  RotationAngle=smiData.RigidTransform(1).angle  RotationAngleUnits=rad  RotationArbitraryAxis=smiData.RigidTransform(1).axis  RotationSequenceAxes=FollowerAxes  RotationSequence=XYX  RotationSequenceAngles=[0 0 0]  RotationSequenceAnglesUnits=deg  RotationMatrix=[1 0 0; 0 1 0; 0 0 1]  Quaternion=[1 0 0 0]  TranslationMethod=Cartesian  TranslationCartesianOffset=smiData.RigidTransform(1).translation  TranslationCartesianOffsetUnits=m  TranslationStandardAxis=+Z  TranslationStandardOffset=0  TranslationStandardOffsetUnits=m  TranslationROffset=0  TranslationROffsetUnits=m  TranslationThetaOffset=0  TranslationThetaOffsetUnits=deg  TranslationZOffset=0  TranslationZOffsetUnits=m
  Transform1 : sm_lib/Frames and Transforms/Rigid Transform  RotationMethod=ArbitraryAxis  FollAlignAxisA=+X  BaseAlignAxisA=+Y  FollAlignAxisB=+Y  BaseAlignAxisB=+Z  RotationStandardAxis=+Z  RotationAngle=smiData.RigidTransform(12).angle  RotationAngleUnits=rad  RotationArbitraryAxis=smiData.RigidTransform(12).axis  RotationSequenceAxes=FollowerAxes  RotationSequence=XYX  RotationSequenceAngles=[0 0 0]  RotationSequenceAnglesUnits=deg  RotationMatrix=[1 0 0; 0 1 0; 0 0 1]  Quaternion=[1 0 0 0]  TranslationMethod=Cartesian  TranslationCartesianOffset=smiData.RigidTransform(12).translation  TranslationCartesianOffsetUnits=m  TranslationStandardAxis=+Z  TranslationStandardOffset=0  TranslationStandardOffsetUnits=m  TranslationROffset=0  TranslationROffsetUnits=m  TranslationThetaOffset=0  TranslationThetaOffsetUnits=deg  TranslationZOffset=0  TranslationZOffsetUnits=m
  F1 : PMIOPort  Side=Left
  F : PMIOPort  Port=2  Side=Right
  connections:
  Solid/RConn1 -- ReferenceFrame/RConn1 -- Transform/LConn1 -- Transform1/LConn1
  Transform/RConn1 -- F/RConn1
  Transform1/RConn1 -- F1/RConn1

== system Forward_and_inverse_Both/6 DOF robot arm/Link4_v2_1_RIGID ==
  ReferenceFrame : sm_lib/Frames and Transforms/Reference Frame
  Solid : sm_lib/Body Elements/File Solid  ExtGeomFileName=C:\Drive D\Material\DC LAB\simscape\simscape\Solidworks FIle\Link4_v2_Default_sldprt.STEP  UnitType=Custom  ExtGeomFileUnits=m  StepReaderType=HEX  ExportConvexHullGeometry=off  InertiaType=Custom  BasedOnType=DensityFromFile  Density=1000  DensityUnits=kg/m^3  Mass=smiData.Solid(4).mass  MassUnits=kg  CenterOfMass=smiData.Solid(4).CoM  CenterOfMassUnits=mm  MomentsOfInertia=smiData.Solid(4).MoI  MomentsOfInertiaUnits=kg*mm^2  ProductsOfInertia=smiData.Solid(4).PoI  ProductsOfInertiaUnits=kg*mm^2  GraphicType=FromGeometry  MarkerShape=Sphere  MarkerSize=10  GraphicVisPropType=SimpleVisualProperties  GraphicDiffuseColor=[0.0 0.8 0.8]  GraphicOpacity=smiData.Solid(4).opacity  GraphicSpecularColor=[0.5 0.5 0.5 1.0]  GraphicAmbientColor=[0.15 0.15 0.15 1.0]  GraphicEmissiveColor=[0.0 0.0 0.0 1.0]  GraphicShininess=75  DoExposeReferenceFrame=on  SerializedFrames=<Frames/>
  Transform : sm_lib/Frames and Transforms/Rigid Transform  RotationMethod=ArbitraryAxis  FollAlignAxisA=+X  BaseAlignAxisA=+Y  FollAlignAxisB=+Y  BaseAlignAxisB=+Z  RotationStandardAxis=+Z  RotationAngle=smiData.RigidTransform(2).angle  RotationAngleUnits=rad  RotationArbitraryAxis=smiData.RigidTransform(2).axis  RotationSequenceAxes=FollowerAxes  RotationSequence=XYX  RotationSequenceAngles=[0 0 0]  RotationSequenceAnglesUnits=deg  RotationMatrix=[1 0 0; 0 1 0; 0 0 1]  Quaternion=[1 0 0 0]  TranslationMethod=Cartesian  TranslationCartesianOffset=smiData.RigidTransform(2).translation  TranslationCartesianOffsetUnits=m  TranslationStandardAxis=+Z  TranslationStandardOffset=0  TranslationStandardOffsetUnits=m  TranslationROffset=0  TranslationROffsetUnits=m  TranslationThetaOffset=0  TranslationThetaOffsetUnits=deg  TranslationZOffset=0  TranslationZOffsetUnits=m
  Transform1 : sm_lib/Frames and Transforms/Rigid Transform  RotationMethod=ArbitraryAxis  FollAlignAxisA=+X  BaseAlignAxisA=+Y  FollAlignAxisB=+Y  BaseAlignAxisB=+Z  RotationStandardAxis=+Z  RotationAngle=smiData.RigidTransform(3).angle  RotationAngleUnits=rad  RotationArbitraryAxis=smiData.RigidTransform(3).axis  RotationSequenceAxes=FollowerAxes  RotationSequence=XYX  RotationSequenceAngles=[0 0 0]  RotationSequenceAnglesUnits=deg  RotationMatrix=[1 0 0; 0 1 0; 0 0 1]  Quaternion=[1 0 0 0]  TranslationMethod=Cartesian  TranslationCartesianOffset=smiData.RigidTransform(3).translation  TranslationCartesianOffsetUnits=m  TranslationStandardAxis=+Z  TranslationStandardOffset=0  TranslationStandardOffsetUnits=m  TranslationROffset=0  TranslationROffsetUnits=m  TranslationThetaOffset=0  TranslationThetaOffsetUnits=deg  TranslationZOffset=0  TranslationZOffsetUnits=m
  F : PMIOPort  Side=Left
  F1 : PMIOPort  Port=2  Side=Right
  connections:
  Solid/RConn1 -- ReferenceFrame/RConn1 -- Transform/LConn1 -- Transform1/LConn1
  Transform/RConn1 -- F/RConn1
  Transform1/RConn1 -- F1/RConn1

== system Forward_and_inverse_Both/6 DOF robot arm/Link5_v2_1_RIGID ==
  ReferenceFrame : sm_lib/Frames and Transforms/Reference Frame
  Solid : sm_lib/Body Elements/File Solid  ExtGeomFileName=C:\Drive D\Material\DC LAB\simscape\simscape\Solidworks FIle\Link5_v2_Default_sldprt.STEP  UnitType=Custom  ExtGeomFileUnits=m  StepReaderType=HEX  ExportConvexHullGeometry=off  InertiaType=Custom  BasedOnType=DensityFromFile  Density=1000  DensityUnits=kg/m^3  Mass=smiData.Solid(6).mass  MassUnits=kg  CenterOfMass=smiData.Solid(6).CoM  CenterOfMassUnits=mm  MomentsOfInertia=smiData.Solid(6).MoI  MomentsOfInertiaUnits=kg*mm^2  ProductsOfInertia=smiData.Solid(6).PoI  ProductsOfInertiaUnits=kg*mm^2  GraphicType=FromGeometry  MarkerShape=Sphere  MarkerSize=10  GraphicVisPropType=SimpleVisualProperties  GraphicDiffuseColor=[0.0 0.8 0.8]  GraphicOpacity=smiData.Solid(6).opacity  GraphicSpecularColor=[0.5 0.5 0.5 1.0]  GraphicAmbientColor=[0.15 0.15 0.15 1.0]  GraphicEmissiveColor=[0.0 0.0 0.0 1.0]  GraphicShininess=75  DoExposeReferenceFrame=on  SerializedFrames=<Frames/>
  Transform : sm_lib/Frames and Transforms/Rigid Transform  RotationMethod=ArbitraryAxis  FollAlignAxisA=+X  BaseAlignAxisA=+Y  FollAlignAxisB=+Y  BaseAlignAxisB=+Z  RotationStandardAxis=+Z  RotationAngle=smiData.RigidTransform(4).angle  RotationAngleUnits=rad  RotationArbitraryAxis=smiData.RigidTransform(4).axis  RotationSequenceAxes=FollowerAxes  RotationSequence=XYX  RotationSequenceAngles=[0 0 0]  RotationSequenceAnglesUnits=deg  RotationMatrix=[1 0 0; 0 1 0; 0 0 1]  Quaternion=[1 0 0 0]  TranslationMethod=Cartesian  TranslationCartesianOffset=smiData.RigidTransform(4).translation  TranslationCartesianOffsetUnits=m  TranslationStandardAxis=+Z  TranslationStandardOffset=0  TranslationStandardOffsetUnits=m  TranslationROffset=0  TranslationROffsetUnits=m  TranslationThetaOffset=0  TranslationThetaOffsetUnits=deg  TranslationZOffset=0  TranslationZOffsetUnits=m
  Transform1 : sm_lib/Frames and Transforms/Rigid Transform  RotationMethod=ArbitraryAxis  FollAlignAxisA=+X  BaseAlignAxisA=+Y  FollAlignAxisB=+Y  BaseAlignAxisB=+Z  RotationStandardAxis=+Z  RotationAngle=smiData.RigidTransform(9).angle  RotationAngleUnits=rad  RotationArbitraryAxis=smiData.RigidTransform(9).axis  RotationSequenceAxes=FollowerAxes  RotationSequence=XYX  RotationSequenceAngles=[0 0 0]  RotationSequenceAnglesUnits=deg  RotationMatrix=[1 0 0; 0 1 0; 0 0 1]  Quaternion=[1 0 0 0]  TranslationMethod=Cartesian  TranslationCartesianOffset=smiData.RigidTransform(9).translation  TranslationCartesianOffsetUnits=m  TranslationStandardAxis=+Z  TranslationStandardOffset=0  TranslationStandardOffsetUnits=m  TranslationROffset=0  TranslationROffsetUnits=m  TranslationThetaOffset=0  TranslationThetaOffsetUnits=deg  TranslationZOffset=0  TranslationZOffsetUnits=m
  F : PMIOPort  Side=Left
  F1 : PMIOPort  Port=2  Side=Right
  connections:
  Solid/RConn1 -- ReferenceFrame/RConn1 -- Transform/LConn1 -- Transform1/LConn1
  Transform/RConn1 -- F/RConn1
  Transform1/RConn1 -- F1/RConn1

== system Forward_and_inverse_Both/6 DOF robot arm2/Base_2_RIGID ==
  ReferenceFrame : sm_lib/Frames and Transforms/Reference Frame
  Solid : sm_lib/Body Elements/File Solid  ExtGeomFileName=C:\Drive D\Material\DC LAB\simscape\simscape\Solidworks FIle\Base_Default_sldprt.STEP  UnitType=Custom  ExtGeomFileUnits=m  StepReaderType=HEX  ExportConvexHullGeometry=off  InertiaType=Custom  BasedOnType=DensityFromFile  Density=1000  DensityUnits=kg/m^3  Mass=smiData.Solid(1).mass  MassUnits=kg  CenterOfMass=smiData.Solid(1).CoM  CenterOfMassUnits=mm  MomentsOfInertia=smiData.Solid(1).MoI  MomentsOfInertiaUnits=kg*mm^2  ProductsOfInertia=smiData.Solid(1).PoI  ProductsOfInertiaUnits=kg*mm^2  GraphicType=FromGeometry  MarkerShape=Sphere  MarkerSize=10  GraphicVisPropType=SimpleVisualProperties  GraphicDiffuseColor=smiData.Solid(1).color  GraphicOpacity=smiData.Solid(1).opacity  GraphicSpecularColor=[0.5 0.5 0.5 1.0]  GraphicAmbientColor=[0.15 0.15 0.15 1.0]  GraphicEmissiveColor=[0.0 0.0 0.0 1.0]  GraphicShininess=75  DoExposeReferenceFrame=on  SerializedFrames=<Frames/>
  Transform : sm_lib/Frames and Transforms/Rigid Transform  RotationMethod=ArbitraryAxis  FollAlignAxisA=+X  BaseAlignAxisA=+Y  FollAlignAxisB=+Y  BaseAlignAxisB=+Z  RotationStandardAxis=+Z  RotationAngle=smiData.RigidTransform(5).angle  RotationAngleUnits=rad  RotationArbitraryAxis=smiData.RigidTransform(5).axis  RotationSequenceAxes=FollowerAxes  RotationSequence=XYX  RotationSequenceAngles=[0 0 0]  RotationSequenceAnglesUnits=deg  RotationMatrix=[1 0 0; 0 1 0; 0 0 1]  Quaternion=[1 0 0 0]  TranslationMethod=Cartesian  TranslationCartesianOffset=smiData.RigidTransform(5).translation  TranslationCartesianOffsetUnits=m  TranslationStandardAxis=+Z  TranslationStandardOffset=0  TranslationStandardOffsetUnits=m  TranslationROffset=0  TranslationROffsetUnits=m  TranslationThetaOffset=0  TranslationThetaOffsetUnits=deg  TranslationZOffset=0  TranslationZOffsetUnits=m
  F1 : PMIOPort  Side=Left
  F : PMIOPort  Port=2  Side=Right
  connections:
  Transform/RConn1 -- F/RConn1
  F1/RConn1 -- Transform/LConn1 -- ReferenceFrame/RConn1 -- Solid/RConn1

== system Forward_and_inverse_Both/6 DOF robot arm2/L1_v2_1_RIGID ==
  ReferenceFrame : sm_lib/Frames and Transforms/Reference Frame
  Solid : sm_lib/Body Elements/File Solid  ExtGeomFileName=C:\Drive D\Material\DC LAB\simscape\simscape\Solidworks FIle\L1_v2_Default_sldprt.STEP  UnitType=Custom  ExtGeomFileUnits=m  StepReaderType=HEX  ExportConvexHullGeometry=off  InertiaType=Custom  BasedOnType=DensityFromFile  Density=1000  DensityUnits=kg/m^3  Mass=smiData.Solid(5).mass  MassUnits=kg  CenterOfMass=smiData.Solid(5).CoM  CenterOfMassUnits=mm  MomentsOfInertia=smiData.Solid(5).MoI  MomentsOfInertiaUnits=kg*mm^2  ProductsOfInertia=smiData.Solid(5).PoI  ProductsOfInertiaUnits=kg*mm^2  GraphicType=FromGeometry  MarkerShape=Sphere  MarkerSize=10  GraphicVisPropType=SimpleVisualProperties  GraphicDiffuseColor=[0.0 0.8 0.8]  GraphicOpacity=smiData.Solid(5).opacity  GraphicSpecularColor=[0.5 0.5 0.5 1.0]  GraphicAmbientColor=[0.15 0.15 0.15 1.0]  GraphicEmissiveColor=[0.0 0.0 0.0 1.0]  GraphicShininess=75  DoExposeReferenceFrame=on  SerializedFrames=<Frames/>
  Transform : sm_lib/Frames and Transforms/Rigid Transform  RotationMethod=ArbitraryAxis  FollAlignAxisA=+X  BaseAlignAxisA=+Y  FollAlignAxisB=+Y  BaseAlignAxisB=+Z  RotationStandardAxis=+Z  RotationAngle=smiData.RigidTransform(6).angle  RotationAngleUnits=rad  RotationArbitraryAxis=smiData.RigidTransform(6).axis  RotationSequenceAxes=FollowerAxes  RotationSequence=XYX  RotationSequenceAngles=[0 0 0]  RotationSequenceAnglesUnits=deg  RotationMatrix=[1 0 0; 0 1 0; 0 0 1]  Quaternion=[1 0 0 0]  TranslationMethod=Cartesian  TranslationCartesianOffset=smiData.RigidTransform(6).translation  TranslationCartesianOffsetUnits=m  TranslationStandardAxis=+Z  TranslationStandardOffset=0  TranslationStandardOffsetUnits=m  TranslationROffset=0  TranslationROffsetUnits=m  TranslationThetaOffset=0  TranslationThetaOffsetUnits=deg  TranslationZOffset=0  TranslationZOffsetUnits=m
  Transform1 : sm_lib/Frames and Transforms/Rigid Transform  RotationMethod=ArbitraryAxis  FollAlignAxisA=+X  BaseAlignAxisA=+Y  FollAlignAxisB=+Y  BaseAlignAxisB=+Z  RotationStandardAxis=+Z  RotationAngle=smiData.RigidTransform(7).angle  RotationAngleUnits=rad  RotationArbitraryAxis=smiData.RigidTransform(7).axis  RotationSequenceAxes=FollowerAxes  RotationSequence=XYX  RotationSequenceAngles=[0 0 0]  RotationSequenceAnglesUnits=deg  RotationMatrix=[1 0 0; 0 1 0; 0 0 1]  Quaternion=[1 0 0 0]  TranslationMethod=Cartesian  TranslationCartesianOffset=smiData.RigidTransform(7).translation  TranslationCartesianOffsetUnits=m  TranslationStandardAxis=+Z  TranslationStandardOffset=0  TranslationStandardOffsetUnits=m  TranslationROffset=0  TranslationROffsetUnits=m  TranslationThetaOffset=0  TranslationThetaOffsetUnits=deg  TranslationZOffset=0  TranslationZOffsetUnits=m
  F : PMIOPort  Side=Left
  F1 : PMIOPort  Port=2  Side=Right
  connections:
  Transform1/RConn1 -- F1/RConn1
  Transform/RConn1 -- F/RConn1
  Transform1/LConn1 -- Transform/LConn1 -- ReferenceFrame/RConn1 -- Solid/RConn1

== system Forward_and_inverse_Both/6 DOF robot arm2/L2_v4_1_RIGID ==
  ReferenceFrame : sm_lib/Frames and Transforms/Reference Frame
  Solid : sm_lib/Body Elements/File Solid  ExtGeomFileName=C:\Drive D\Material\DC LAB\simscape\simscape\Solidworks FIle\L2_v4_Default_sldprt.STEP  UnitType=Custom  ExtGeomFileUnits=m  StepReaderType=HEX  ExportConvexHullGeometry=off  InertiaType=Custom  BasedOnType=DensityFromFile  Density=1000  DensityUnits=kg/m^3  Mass=smiData.Solid(3).mass  MassUnits=kg  CenterOfMass=smiData.Solid(3).CoM  CenterOfMassUnits=mm  MomentsOfInertia=smiData.Solid(3).MoI  MomentsOfInertiaUnits=kg*mm^2  ProductsOfInertia=smiData.Solid(3).PoI  ProductsOfInertiaUnits=kg*mm^2  GraphicType=FromGeometry  MarkerShape=Sphere  MarkerSize=10  GraphicVisPropType=SimpleVisualProperties  GraphicDiffuseColor=[0.0 0.8 0.8]  GraphicOpacity=smiData.Solid(3).opacity  GraphicSpecularColor=[0.5 0.5 0.5 1.0]  GraphicAmbientColor=[0.15 0.15 0.15 1.0]  GraphicEmissiveColor=[0.0 0.0 0.0 1.0]  GraphicShininess=75  DoExposeReferenceFrame=on  SerializedFrames=<Frames/>
  Transform : sm_lib/Frames and Transforms/Rigid Transform  RotationMethod=ArbitraryAxis  FollAlignAxisA=+X  BaseAlignAxisA=+Y  FollAlignAxisB=+Y  BaseAlignAxisB=+Z  RotationStandardAxis=+Z  RotationAngle=smiData.RigidTransform(8).angle  RotationAngleUnits=rad  RotationArbitraryAxis=smiData.RigidTransform(8).axis  RotationSequenceAxes=FollowerAxes  RotationSequence=XYX  RotationSequenceAngles=[0 0 0]  RotationSequenceAnglesUnits=deg  RotationMatrix=[1 0 0; 0 1 0; 0 0 1]  Quaternion=[1 0 0 0]  TranslationMethod=Cartesian  TranslationCartesianOffset=smiData.RigidTransform(8).translation  TranslationCartesianOffsetUnits=m  TranslationStandardAxis=+Z  TranslationStandardOffset=0  TranslationStandardOffsetUnits=m  TranslationROffset=0  TranslationROffsetUnits=m  TranslationThetaOffset=0  TranslationThetaOffsetUnits=deg  TranslationZOffset=0  TranslationZOffsetUnits=m
  Transform1 : sm_lib/Frames and Transforms/Rigid Transform  RotationMethod=ArbitraryAxis  FollAlignAxisA=+X  BaseAlignAxisA=+Y  FollAlignAxisB=+Y  BaseAlignAxisB=+Z  RotationStandardAxis=+Z  RotationAngle=smiData.RigidTransform(11).angle  RotationAngleUnits=rad  RotationArbitraryAxis=smiData.RigidTransform(11).axis  RotationSequenceAxes=FollowerAxes  RotationSequence=XYX  RotationSequenceAngles=[0 0 0]  RotationSequenceAnglesUnits=deg  RotationMatrix=[1 0 0; 0 1 0; 0 0 1]  Quaternion=[1 0 0 0]  TranslationMethod=Cartesian  TranslationCartesianOffset=smiData.RigidTransform(11).translation  TranslationCartesianOffsetUnits=m  TranslationStandardAxis=+Z  TranslationStandardOffset=0  TranslationStandardOffsetUnits=m  TranslationROffset=0  TranslationROffsetUnits=m  TranslationThetaOffset=0  TranslationThetaOffsetUnits=deg  TranslationZOffset=0  TranslationZOffsetUnits=m
  F : PMIOPort  Side=Left
  F1 : PMIOPort  Port=2  Side=Right
  connections:
  Transform1/RConn1 -- F1/RConn1
  Transform/RConn1 -- F/RConn1
  Transform1/LConn1 -- Transform/LConn1 -- ReferenceFrame/RConn1 -- Solid/RConn1

== system Forward_and_inverse_Both/6 DOF robot arm2/L6_2_RIGID ==
  ReferenceFrame : sm_lib/Frames and Transforms/Reference Frame
  Solid : sm_lib/Body Elements/File Solid  ExtGeomFileName=C:\Drive D\Material\DC LAB\simscape\simscape\Solidworks FIle\L6_Default_sldprt.STEP  UnitType=Custom  ExtGeomFileUnits=m  StepReaderType=HEX  ExportConvexHullGeometry=off  InertiaType=Custom  BasedOnType=DensityFromFile  Density=1000  DensityUnits=kg/m^3  Mass=smiData.Solid(7).mass  MassUnits=kg  CenterOfMass=smiData.Solid(7).CoM  CenterOfMassUnits=mm  MomentsOfInertia=smiData.Solid(7).MoI  MomentsOfInertiaUnits=kg*mm^2  ProductsOfInertia=smiData.Solid(7).PoI  ProductsOfInertiaUnits=kg*mm^2  GraphicType=FromGeometry  MarkerShape=Sphere  MarkerSize=10  GraphicVisPropType=SimpleVisualProperties  GraphicDiffuseColor=[0.0 0.8 0.8]  GraphicOpacity=smiData.Solid(7).opacity  GraphicSpecularColor=[0.5 0.5 0.5 1.0]  GraphicAmbientColor=[0.15 0.15 0.15 1.0]  GraphicEmissiveColor=[0.0 0.0 0.0 1.0]  GraphicShininess=75  DoExposeReferenceFrame=on  SerializedFrames=<Frames/>
  Transform : sm_lib/Frames and Transforms/Rigid Transform  RotationMethod=ArbitraryAxis  FollAlignAxisA=+X  BaseAlignAxisA=+Y  FollAlignAxisB=+Y  BaseAlignAxisB=+Z  RotationStandardAxis=+Z  RotationAngle=smiData.RigidTransform(10).angle  RotationAngleUnits=rad  RotationArbitraryAxis=smiData.RigidTransform(10).axis  RotationSequenceAxes=FollowerAxes  RotationSequence=XYX  RotationSequenceAngles=[0 0 0]  RotationSequenceAnglesUnits=deg  RotationMatrix=[1 0 0; 0 1 0; 0 0 1]  Quaternion=[1 0 0 0]  TranslationMethod=Cartesian  TranslationCartesianOffset=smiData.RigidTransform(10).translation  TranslationCartesianOffsetUnits=m  TranslationStandardAxis=+Z  TranslationStandardOffset=0  TranslationStandardOffsetUnits=m  TranslationROffset=0  TranslationROffsetUnits=m  TranslationThetaOffset=0  TranslationThetaOffsetUnits=deg  TranslationZOffset=0  TranslationZOffsetUnits=m
  F : PMIOPort  Side=Left
  connections:
  Transform/RConn1 -- F/RConn1
  Transform/LConn1 -- ReferenceFrame/RConn1 -- Solid/RConn1
